simulink model "sender"  (R2022a)
settings: Solver=FixedStepDiscrete  StartTime=0.0  StopTime=inf  RelTol=1e-3
libraries: androiduilib x5, androidaudiovideolib x2, androidcommunicationlib x2
settings Model: Creator=GautamVashishtha  LastModifiedBy=GautamVashishtha
settings OptimizationCC: EnhancedBackFolding=on  PassReuseOutputArgsAs=Individual arguments  ZeroExternalMemoryAtStartup=off  ZeroInternalMemoryAtStartup=off  MaxStackSize=64  OptimizeBlockOrder=speed  DifferentSizesBufferReuse=on  OptimizationCustomize=off  EfficientTunableParamExpr=on
settings DebuggingCC: ParameterTunabilityLossMsg=error
settings HardwareCC: ProdBitPerPointer=32  ProdBitPerSizeT=32  ProdBitPerPtrDiffT=32  ProdLargestAtomicInteger=Long  ProdLargestAtomicFloat=Double  ProdWordSize=32  ProdHWDeviceType=ARM Compatible->ARM Cortex  UseEmbeddedCoderFeatures=off  UseSimulinkCoderFeatures=off
settings SFSimCC: MATLABDynamicMemAlloc=off
settings RTWCC: SystemTargetFile=ert.tlc  HardwareBoard=Android Device  TLCOptions="-aInlineSetEventsForThisBaseRateFcn=TLC_FALSE -aSuppressMultiTaskScheduler=TLC_FALSE  -aRateBasedStepFcn=0"  TemplateMakefile=ert_default_tmf  RTWVerbose=off  Toolchain=Android SDK/NDK Tools
settings CodeAppCC: ForceParamTrailComments=on  IgnoreCustomStorageClasses=off  OperatorAnnotations=on  SimulinkDataObjDesc=on  SFDataObjDesc=on  InsertBlockDesc=on
settings ERTTargetCC: SupportNonInlinedSFcns=on

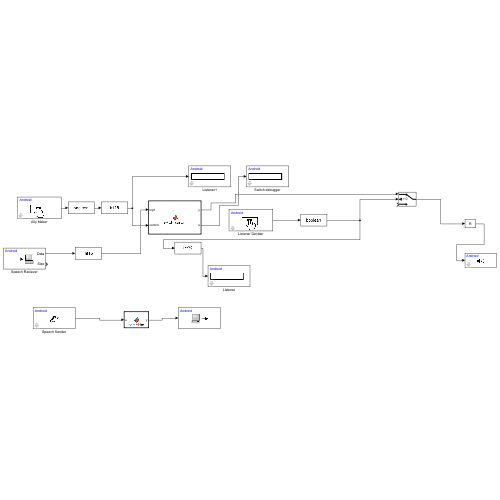
[thumbnail: Simulink's stored preview of the top-level diagram]
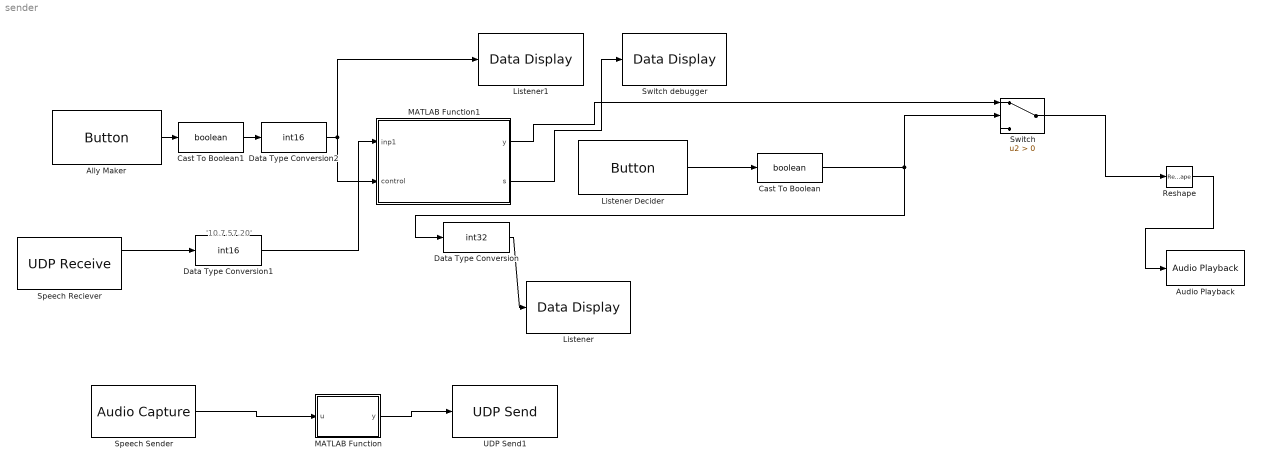
== system sender ==
  note: '10.7.57.20'
  Ally Maker : androiduilib/Button  ButtonState=Not pressed  ButtonId=sender/Ally_Maker  State=off  SampleTime=0.1  BlockPlatform=Android
      settings: SourceProductBaseCode=ANDROID
  Audio Playback : androidaudiovideolib/Audio Playback  SampleFreq=44100  AudioSamplingFreq=44100  SampleTime=0.1  DeviceStr=0  QueueDuration=0  BlockPlatform=Android
      settings: SourceProductBaseCode=ANDROID
  Cast To Boolean : DataTypeConversion  OutDataTypeStr=boolean  SaturateOnIntegerOverflow=off  RndMeth=Floor
  Cast To Boolean1 : DataTypeConversion  OutDataTypeStr=boolean  SaturateOnIntegerOverflow=off  RndMeth=Floor
  Data Type Conversion : DataTypeConversion  OutDataTypeStr=int32  SaturateOnIntegerOverflow=off  RndMeth=Floor
  Data Type Conversion1 : DataTypeConversion  OutDataTypeStr=int16  SaturateOnIntegerOverflow=off  RndMeth=Floor
  Data Type Conversion2 : DataTypeConversion  OutDataTypeStr=int16  SaturateOnIntegerOverflow=off  RndMeth=Floor
  Listener : androiduilib/Data Display  DataDisplayId=sender/Listener  Format=Integer  Precision=6  SimulateUsing=Code generation  blockPlatform=Android
      settings: SourceProductBaseCode=ANDROID
  Listener Decider : androiduilib/Button  ButtonState=Not pressed  ButtonId=sender/Listener_Decider  State=off  SampleTime=0.1  BlockPlatform=Android
      settings: SourceProductBaseCode=ANDROID
  Listener1 : androiduilib/Data Display  DataDisplayId=sender/Listener1  Format=Integer  Precision=6  SimulateUsing=Code generation  blockPlatform=Android
      settings: SourceProductBaseCode=ANDROID
  MATLAB Function : MATLAB Function  TreatAsAtomicUnit=on
  MATLAB Function1 : MATLAB Function  TreatAsAtomicUnit=on
  Reshape : Reshape  OutputDimensionality=Customize  OutputDimensions=[4410,2]
  Speech Reciever : androidcommunicationlib/UDP Receive  localURL='0.0.0.0'  localPort=8000  remoteURL='0.0.0.0'  remotePort=-1  recvBufferSize=8192  signalDatatype=int16  dims=8820  isVarSize=off  showBlockingTime=off  blockingTime=0  sampletime=0.1  blockPlatform=Android
      settings: SourceProductBaseCode=ANDROID
  Speech Sender : androidaudiovideolib/Audio Capture  SampleFreq=44100  FrameSize=4410  SampleTime=0.1  SimulateUsing=Code generation  DeviceStr=0  QueueDuration=0  BlockPlatform=Android  AudioSamplingFreq=44100
      settings: SourceProductBaseCode=ANDROID
  Switch : Switch  Criteria=u2 > Threshold  SaturateOnIntegerOverflow=off  InputSameDT=off
  Switch debugger : androiduilib/Data Display  DataDisplayId=sender/Switch_debugger  Format=Integer  Precision=6  SimulateUsing=Code generation  blockPlatform=Android
      settings: SourceProductBaseCode=ANDROID
  UDP Send1 : androidcommunicationlib/UDP Send  remoteURL='10.7.56.158'  remotePort=8000  localURL='0.0.0.0'  localPortSource=Automatically determine  localPort=-1  sampletime=-1  blockPlatform=Android  separateLengthPort=0
      settings: SourceProductBaseCode=ANDROID
  wires:
  Data Type Conversion/1 -> Listener/1
  Speech Sender/1 -> MATLAB Function/1(u)
  Cast To Boolean1/1 -> Data Type Conversion2/1
  Ally Maker/1 -> Cast To Boolean1/1
  Listener Decider/1 -> Cast To Boolean/1
  Speech Reciever/1 -> Data Type Conversion1/1
  Data Type Conversion2/1 -> Listener1/1, MATLAB Function1/2(control)
  Cast To Boolean/1 -> Data Type Conversion/1, Switch/2
  MATLAB Function1/2(s) -> Switch debugger/1
  MATLAB Function/1(y) -> UDP Send1/1
  Switch/1 -> Reshape/1
  Reshape/1 -> Audio Playback/1
  MATLAB Function1/1(y) -> Switch/1
  Data Type Conversion1/1 -> MATLAB Function1/1(inp1)

== matlab function sender/MATLAB Function1 ==
  data: inp1 input; y output; control input; s output
function [y,s] = switch_custom(inp1,control)


if control==1
%     UnScramble the input
    y = flip(inp1);
    s  = 1;
else
    
    y = inp1;
    s  = 2;
end

== matlab function sender/MATLAB Function ==
  data: u input; y output
function y = scrambler(u)
y = flip(u);
